simulink model "RCpulseSIM"  (R2013b)
settings: Solver=ode3  SolverMode=SingleTasking  StartTime=0.0  StopTime=10  RelTol=1e-3
undefined symbols (not defined in the file): Ts
libraries: arduino_io_lib x4
settings Model: ExtModeTrigDuration=2  Creator=gcampa  LastModifiedBy=richard.hill
settings OptimizationCC: OptimizeModelRefInitCode=on  LifeSpan=1
settings DebuggingCC: SolverPrmCheckMsg=none
settings HardwareCC: ProdBitPerInt=16  ProdBitPerPointer=8  ProdIntDivRoundTo=Zero  ProdEndianess=LittleEndian  ProdWordSize=8  ProdHWDeviceType=Atmel->AVR
settings RTWCC: SystemTargetFile=realtime.tlc  GenerateMakefile=off  TemplateMakefile=realtime.tmf  Description=Run on Target Hardware  RTWVerbose=off  ProcessScript=realtime_make_rtw_hook
settings STFCustomTargetCC: TargetLibSuffix=.a  CodeReplacementLibrary=None  GenerateSampleERTMain=on  ERTCustomFileBanners=on  SupportNonInlinedSFcns=off  SupportVariableSizeSignals=on  MATLABClassNameForMDSCustomization=Simulink.SoftwareTarget.ERTCustomization  GRTInterface=off  SystemTargetFile=realtime.tlc
settings ERTTargetCC: GenerateSampleERTMain=on  ParMdlRefBuildCompliant=off  CompOptLevelCompliant=off  ConcurrentExecutionCompliant=off  CombineOutputUpdateFcns=off  ERTFirstTimeCompliant=off  SupportContinuousTime=on  SupportVariableSizeSignals=on  ModelStepFunctionPrototypeControlCompliant=off  CPPClassGenCompliant=off  ExtModeTransport=3  ExtModeMexFile=ext_serial_win32_comm  ExtModeMexArgs=0 1 9600  InlinedParameterPlacement=NonHierarchical  ERTSrcFileBannerTemplate=realtime_code_template.cgt  ERTHdrFileBannerTemplate=realtime_code_template.cgt  ERTDataSrcFileTemplate=realtime_code_template.cgt  ERTDataHdrFileTemplate=realtime_code_template.cgt  ERTCustomFileTemplate=realtime_file_process.tlc

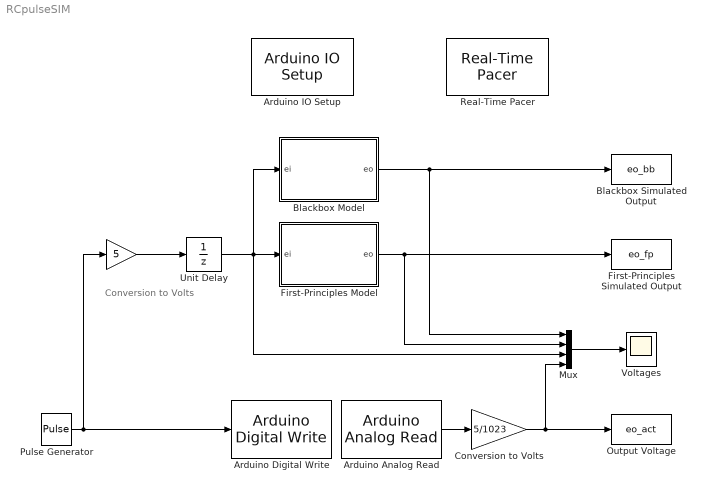
== system RCpulseSIM ==
  note: Conversion
      | to Volts
  " " : Gain  Gain=5
  Arduino Analog Read : arduino_io_lib/Arduino Analog Read  arduinoVar=Temporary arduino variable: Arduino1  arduinoPin=0  T=Ts
  Arduino Digital Write : arduino_io_lib/Arduino Digital Write  arduinoVar=Temporary arduino variable: Arduino1  arduinoPin=8  T=-1
  Arduino IO Setup : arduino_io_lib/Arduino IO Setup  Priority=3  arduinoVar=Temporary arduino variable: Arduino1  workspaceVarName=b  comPort=COM5
  Blackbox Model : Subsystem  mask{K=1, tau=1.06}
      mask prompts: K "DC gain"; tau "Time constant"
      mask Display:
      | port_label('input',1,'ei')
      | port_label('output',1,'eo')
  Blackbox Simulated Output : ToWorkspace  VariableName=eo_bb  SampleTime=-1
  Conversion to Volts : Gain  Gain=5/1023
  First-Principles Simulated Output : ToWorkspace  VariableName=eo_fp  SampleTime=-1
  First-Principles Model : Subsystem  mask{R=9840, C=103.4*10^-6, q_init=0}
      mask prompts: R "Resistance"; C "Capacitance"; q_init "Initial charge on capacitor"
      mask Display:
      | port_label('input',1,'ei')
      | port_label('output',1,'eo')
  Mux : Mux
  Output Voltage : ToWorkspace  VariableName=eo_act  SampleTime=-1
  Pulse Generator : DiscretePulseGenerator  Period=100  PulseWidth=50  PhaseDelay=50  SampleTime=Ts
  Real-Time Pacer : arduino_io_lib/Real-Time Pacer  simTimePerRealTime=1
  Unit Delay : UnitDelay  SampleTime=-1
  Voltages : Scope
  wires:
  Arduino Analog Read/1 -> Conversion to Volts/1
  Mux/1 -> Voltages/1
  Conversion to Volts/1 -> Mux/4, Output Voltage/1
  First-Principles Model/1(eo) -> First-Principles Simulated Output/1, Mux/2
  " "/1 -> Unit Delay/1
  Pulse Generator/1 -> " "/1, Arduino Digital Write/1
  Blackbox Model/1(eo) -> Mux/1, Blackbox Simulated Output/1
  Unit Delay/1 -> Blackbox Model/1(ei), First-Principles Model/1(ei), Mux/3

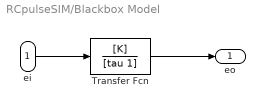
== system RCpulseSIM/Blackbox Model ==
  ei : Inport
  Transfer Fcn : TransferFcn  Numerator=[K]  Denominator=[tau 1]
  eo : Outport
  wires:
  ei/1 -> Transfer Fcn/1
  Transfer Fcn/1 -> eo/1

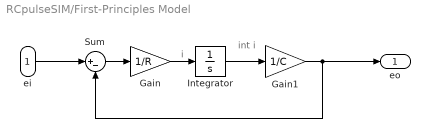
== system RCpulseSIM/First-Principles Model ==
  note: int i
  note: i
  ei : Inport
  Gain : Gain  Gain=1/R  SampleTime=0.1
  Gain1 : Gain  Gain=1/C  SampleTime=0.1
  Integrator : Integrator  InitialCondition=q_init
  Sum : Sum  Inputs=|+-
  eo : Outport
  wires:
  Gain/1 -> Integrator/1
  Sum/1 -> Gain/1
  Integrator/1 -> Gain1/1
  Gain1/1 -> Sum/2, eo/1
  ei/1 -> Sum/1
